simulink model "double_link_lqr"  (R2026a)
settings: Solver=ode45  StopTime=sim_time
undefined symbols (not defined in the file): A, B, C, D, K, u_max, x0
settings Model: Creator=H.Tam  LastModifiedBy=H.Tam

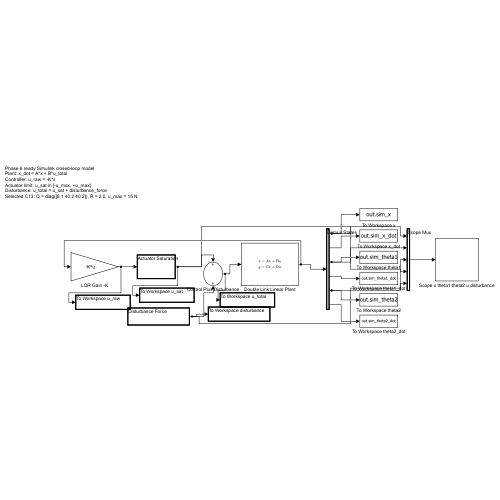
[thumbnail: Simulink's stored preview of the top-level diagram]
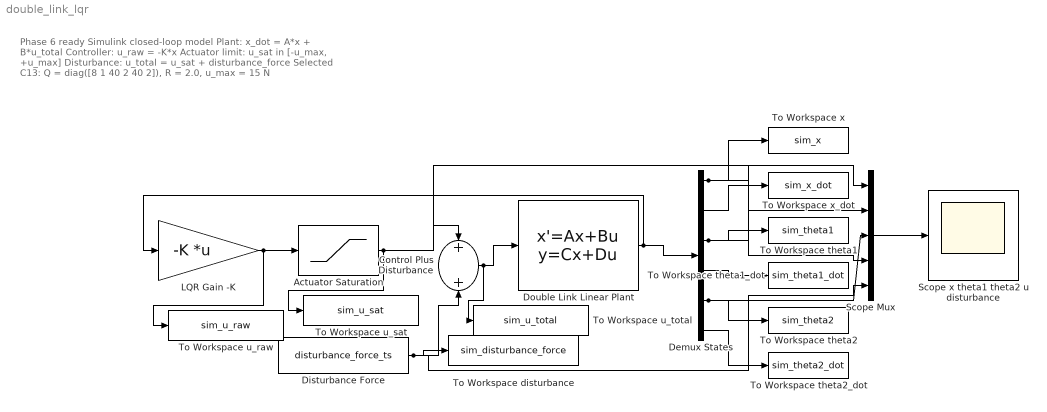
== system double_link_lqr ==
  note: Phase 6 ready Simulink closed-loop model
      | Plant: x_dot = A*x + B*u_total
      | Controller: u_raw = -K*x
      | Actuator limit: u_sat in [-u_max, +u_max]
      | Disturbance: u_total = u_sat + disturbance_force
      | Selected C13: Q = diag([8 1 40 2 40 2]), R = 2.0, u_max = 15 N
  Actuator Saturation : Saturate  UpperLimit=u_max  LowerLimit=-u_max
  Control Plus Disturbance : Sum
  Demux States : Demux  Outputs=6
  Disturbance Force : FromWorkspace  VariableName=disturbance_force_ts
  Double Link Linear Plant : StateSpace  A=A  B=B  C=C  D=D  InitialCondition=x0
  LQR Gain -K : Gain  Gain=-K  Multiplication=Matrix(K*u)
  Scope Mux : Mux  Inputs=5
  Scope x theta1 theta2 u disturbance : Scope
  To Workspace disturbance : ToWorkspace  VariableName=sim_disturbance_force  SaveFormat=Structure With Time  SampleTime=-1
  To Workspace theta1 : ToWorkspace  VariableName=sim_theta1  SaveFormat=Structure With Time  SampleTime=-1
  To Workspace theta1_dot : ToWorkspace  VariableName=sim_theta1_dot  SaveFormat=Structure With Time  SampleTime=-1
  To Workspace theta2 : ToWorkspace  VariableName=sim_theta2  SaveFormat=Structure With Time  SampleTime=-1
  To Workspace theta2_dot : ToWorkspace  VariableName=sim_theta2_dot  SaveFormat=Structure With Time  SampleTime=-1
  To Workspace u_raw : ToWorkspace  VariableName=sim_u_raw  SaveFormat=Structure With Time  SampleTime=-1
  To Workspace u_sat : ToWorkspace  VariableName=sim_u_sat  SaveFormat=Structure With Time  SampleTime=-1
  To Workspace u_total : ToWorkspace  VariableName=sim_u_total  SaveFormat=Structure With Time  SampleTime=-1
  To Workspace x : ToWorkspace  VariableName=sim_x  SaveFormat=Structure With Time  SampleTime=-1
  To Workspace x_dot : ToWorkspace  VariableName=sim_x_dot  SaveFormat=Structure With Time  SampleTime=-1
  wires:
  Double Link Linear Plant/1 -> LQR Gain -K/1, Demux States/1
  LQR Gain -K/1 -> Actuator Saturation/1, To Workspace u_raw/1
  Actuator Saturation/1 -> Control Plus Disturbance/1, To Workspace u_sat/1, Scope Mux/4
  Disturbance Force/1 -> Control Plus Disturbance/2, To Workspace disturbance/1, Scope Mux/5
  Control Plus Disturbance/1 -> Double Link Linear Plant/1, To Workspace u_total/1
  Demux States/1 -> To Workspace x/1, Scope Mux/1
  Demux States/2 -> To Workspace x_dot/1
  Demux States/3 -> To Workspace theta1/1, Scope Mux/2
  Demux States/4 -> To Workspace theta1_dot/1
  Demux States/5 -> To Workspace theta2/1, Scope Mux/3
  Demux States/6 -> To Workspace theta2_dot/1
  Scope Mux/1 -> Scope x theta1 theta2 u disturbance/1
